simulink model "adaptive_IMC_cont"  (Simulink 7.0)
settings: Solver=ode4  StartTime=0.0  StopTime=Inf  FixedStep=1  RelTol=1e-3
settings Model: Creator=ismt  LastModifiedBy=ismt

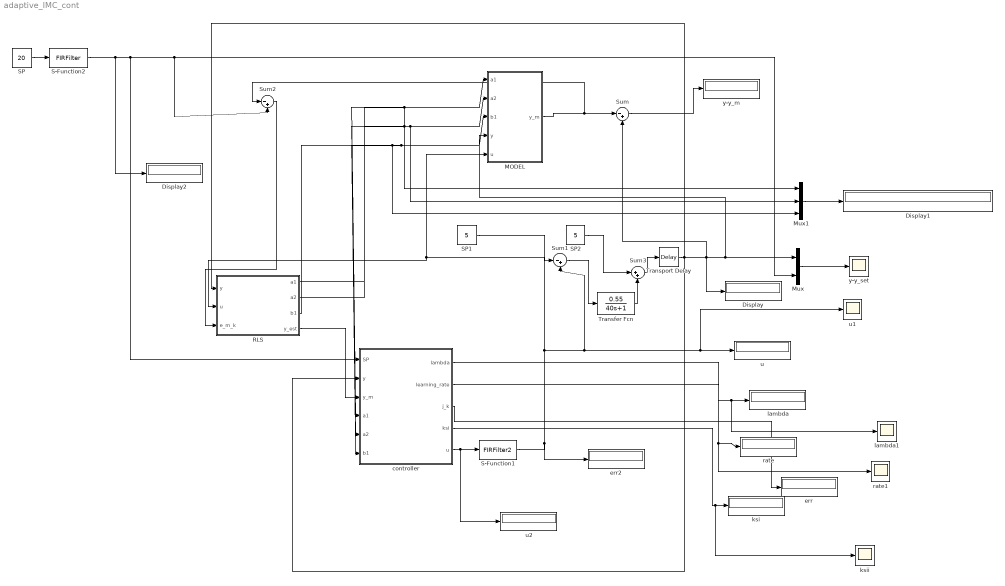
== system adaptive_IMC_cont ==
  Display : Display
  Display1 : Display
  Display2 : Display
  MODEL : Subsystem
  Mux : Mux  Inputs=2
  Mux1 : Mux  Inputs=3
  RLS : Subsystem  mask{a10=0, a20=0, b10=0.01, gamma=1000}
      mask prompts: a10 "a1"; a20 "a2"; b10 "b1"
  S-Function1 : S-Function  FunctionName=FIRFilter2
  S-Function2 : S-Function  FunctionName=FIRFilter
  SP : Constant  Value=20  OutDataType=sfix(16)  OutScaling=2^0
  SP1 : Constant  Value=5  OutDataType=sfix(16)  OutScaling=2^0
  SP2 : Constant  Value=5  OutDataType=sfix(16)  OutScaling=2^0
  Sum : Sum  Inputs=|-+  OutDataType=sfix(16)  OutScaling=2^0
  Sum1 : Sum  Inputs=|-+  OutDataType=sfix(16)  OutScaling=2^0
  Sum2 : Sum  Inputs=|-+  OutDataType=sfix(16)  OutScaling=2^0
  Sum3 : Sum  Inputs=|++  OutDataType=sfix(16)  OutScaling=2^0
  Transfer Fcn : TransferFcn  Numerator=[0.55]  Denominator="[ 40  1]"
  Transport Delay : TransportDelay  DelayTime=2
  controller : Subsystem  mask{ksi0=0.7, n0=1, K=0.05, threshold=1, I_inc=1.005, I_dec=0.999}
      mask prompts: ksi0 "ksi"; n0 "learning_rate"
  err : Display
  err2 : Display
  ksi : Display
  ksii : Scope
      settings: TimeRange=25000  YMin=0.69995  YMax=0.7007  SaveName=ScopeData3
  lambda : Display
  lambda1 : Scope
      settings: TimeRange=9000  YMin=0  YMax=0.9
  rate : Display
  rate1 : Scope
      settings: TimeRange=25000  YMin=0  YMax=55  SaveName=ScopeData2
  u : Display
  u1 : Scope
      settings: TimeRange=2500  YMin=0  YMax=100  SaveName=ScopeData4
  u2 : Display
  y-y_m : Display
  y-y_set : Scope
      settings: TimeRange=25000  YMin=0  YMax=60
  wires:
  SP/1 -> S-Function2/1
  Mux/1 -> y-y_set/1
  RLS/1(a1) -> MODEL/1(a1), Mux1/1, controller/4(a1)
  RLS/2(a2) -> controller/5(a2), MODEL/2(a2), Mux1/2
  RLS/3(b1) -> MODEL/3(b1), controller/6(b1), Mux1/3
  Sum/1 -> y-y_m/1
  Mux1/1 -> Display1/1
  MODEL/1(y_m) -> Sum/1, Sum2/1
  RLS/4(y_est) -> controller/3(y_m)
  controller/5(u) -> S-Function1/1, u2/1
  controller/1(lambda) -> lambda/1, lambda1/1
  controller/2(learning_rate) -> rate/1, rate1/1
  controller/3(j_k) -> err/1
  controller/4(ksi) -> ksi/1, ksii/1
  SP1/1 -> Sum1/1
  Sum2/1 -> RLS/3(e_m_k)
  Sum1/1 -> Transfer Fcn/1
  Transport Delay/1 -> Display/1, Mux/1, MODEL/4(y), Sum/2, RLS/1(y), controller/2(y)
  S-Function1/1 -> Sum1/2, u/1, u1/1, MODEL/5(u), RLS/2(u), err2/1
  S-Function2/1 -> controller/1(SP), Mux/2, Sum2/2, Display2/1
  Transfer Fcn/1 -> Sum3/2
  SP2/1 -> Sum3/1
  Sum3/1 -> Transport Delay/1

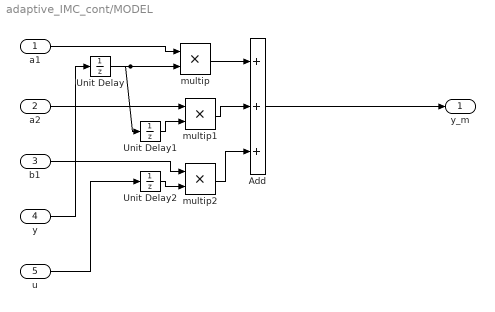
== system adaptive_IMC_cont/MODEL ==
  a1 : Inport
  a2 : Inport  Port=2
  b1 : Inport  Port=3
  y : Inport  Port=4
  u : Inport  Port=5
  Add : Sum  Inputs=+++  OutDataType=sfix(16)  OutScaling=2^-10
  Unit Delay : UnitDelay
  Unit Delay1 : UnitDelay
  Unit Delay2 : UnitDelay
  multip : Product  Inputs=**  OutDataType=sfix(16)  OutScaling=2^-10
  multip1 : Product  Inputs=**  OutDataType=sfix(16)  OutScaling=2^-10
  multip2 : Product  Inputs=**  OutDataType=sfix(16)  OutScaling=2^-10
  y_m : Outport
  wires:
  Add/1 -> y_m/1
  a1/1 -> multip/1
  y/1 -> Unit Delay/1
  Unit Delay/1 -> multip/2, Unit Delay1/1
  multip/1 -> Add/1
  multip1/1 -> Add/2
  a2/1 -> multip1/1
  Unit Delay1/1 -> multip1/2
  u/1 -> Unit Delay2/1
  Unit Delay2/1 -> multip2/2
  multip2/1 -> Add/3
  b1/1 -> multip2/1

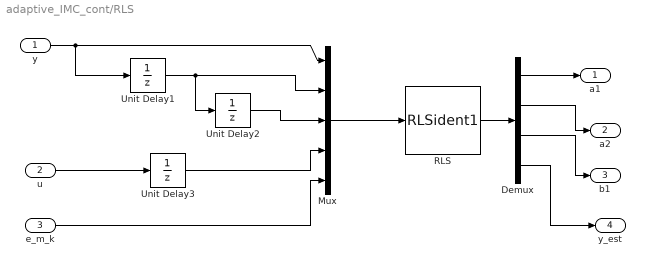
== system adaptive_IMC_cont/RLS ==
  y : Inport
  u : Inport  Port=2
  e_m_k : Inport  Port=3
  Demux : Demux
  Mux : Mux  Inputs=5
  RLS : S-Function  FunctionName=RLSident1  Parameters=a10,a20,b10,gamma
  Unit Delay1 : UnitDelay
  Unit Delay2 : UnitDelay
  Unit Delay3 : UnitDelay
  a1 : Outport
  a2 : Outport  Port=2
  b1 : Outport  Port=3
  y_est : Outport  Port=4
  wires:
  y/1 -> Mux/1, Unit Delay1/1
  Mux/1 -> RLS/1
  Unit Delay1/1 -> Mux/2, Unit Delay2/1
  Unit Delay2/1 -> Mux/3
  u/1 -> Unit Delay3/1
  Unit Delay3/1 -> Mux/4
  RLS/1 -> Demux/1
  Demux/1 -> a1/1
  Demux/4 -> y_est/1
  Demux/3 -> b1/1
  Demux/2 -> a2/1
  e_m_k/1 -> Mux/5

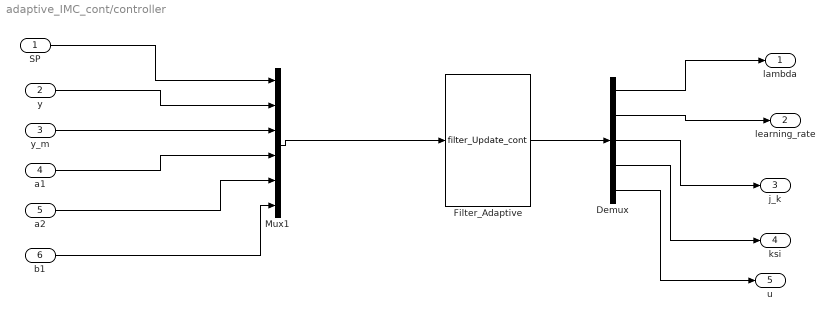
== system adaptive_IMC_cont/controller ==
  SP : Inport
  y : Inport  Port=2
  y_m : Inport  Port=3
  a1 : Inport  Port=4
  a2 : Inport  Port=5
  b1 : Inport  Port=6
  Demux : Demux  Outputs=5
  Filter_Adaptive : S-Function  FunctionName=filter_Update_cont  Parameters=ksi0, n0, K, threshold, I_inc, I_dec
  Mux1 : Mux  Inputs=6
  lambda : Outport
  learning_rate : Outport  Port=2
  j_k : Outport  Port=3
  ksi : Outport  Port=4
  u : Outport  Port=5
  wires:
  SP/1 -> Mux1/1
  y/1 -> Mux1/2
  y_m/1 -> Mux1/3
  a1/1 -> Mux1/4
  a2/1 -> Mux1/5
  b1/1 -> Mux1/6
  Mux1/1 -> Filter_Adaptive/1
  Filter_Adaptive/1 -> Demux/1
  Demux/1 -> lambda/1
  Demux/2 -> learning_rate/1
  Demux/3 -> j_k/1
  Demux/4 -> ksi/1
  Demux/5 -> u/1
